simulink model "consistency"  (R2021a)
settings: Solver=VariableStepAuto  StartTime=0.0001  StopTime=180  FixedStep=0.01  RelTol=1e-6  AbsTol=1e-6
values from neighbouring files (symbols this model uses):
  A = kron(D,kron(B3,(B2*k1+B1*B2')))-kron(L,kron(B3,B2*k2))    [init.m]    (also in main.m)
  A_xi = kron(B3,B2*k1+B1*B2')    [init.m]    (also in main.m)
  B_h = kron(D,kron(B3,B2*k1))-kron(L,kron(B3,B2*k2))    [init.m]    (also in main.m)
  B_hv = kron(D,kron(B3,B2))    [init.m]    (also in main.m)
  B_xi = kron(VV(1,:),kron(B3,B1))    [init.m]    (also in main.m)
  theta0 = [theta10;theta20;theta30;theta40;theta50]    [init.m]    (also in main.m)
  xi0 = kron(VV(1,:),kron(B3,B3))*(theta0-ht0)    [init.m]    (also in main.m)
undefined symbols (not defined in the file or in its folder): dfcn_ht, fcn_ht, fcn_xi
settings Model: Creator=xxx  LastModifiedBy=Alpha
settings SolverCC: AutoScaleAbsTol=off  AlgebraicLoopSolver=TrustRegion
settings DataIOCC: ReturnWorkspaceOutputs=off
settings DebuggingCC: SFMachineParentedDataDiag=warning  ArithmeticOperatorsInVariantConditions=warning
settings SFSimCC: SimUseLocalCustomCode=off  CustomCodeUndefinedFunction=UseInterfaceOnly
settings RTWCC: RTWUseLocalCustomCode=off
settings CodeAppCC: StateflowObjectComments=on

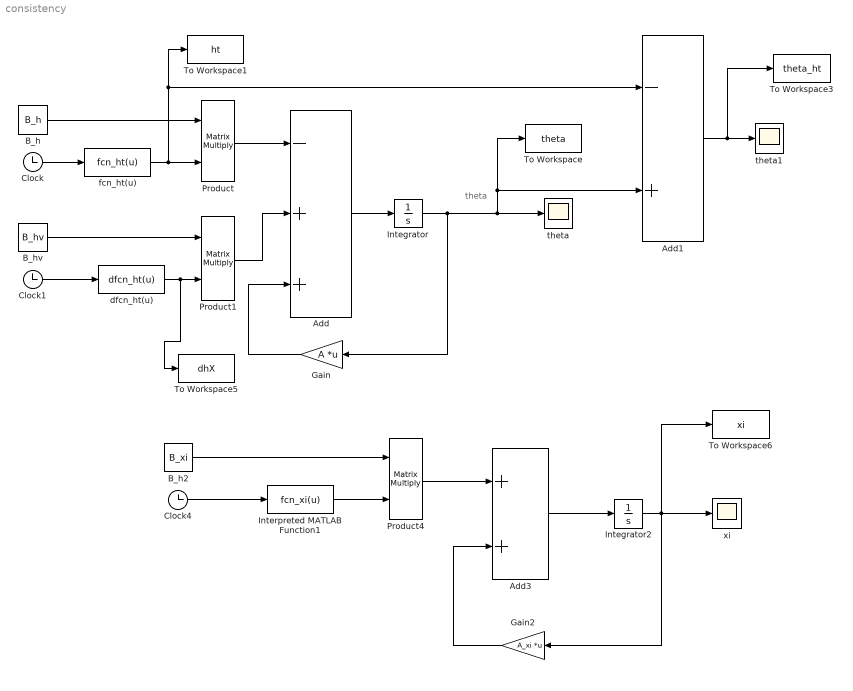
== system consistency ==
  note: theta
  Add : Sum  Inputs=-++
  Add1 : Sum  Inputs=-+
  Add3 : Sum
  B_h : Constant  Value=B_h
  B_h2 : Constant  Value=B_xi
  B_hv : Constant  Value=B_hv
  Clock : Clock
  Clock1 : Clock
  Clock4 : Clock
  Gain : Gain  Gain=A  Multiplication=Matrix(K*u)
  Gain2 : Gain  Gain=A_xi  Multiplication=Matrix(K*u)
  Integrator : Integrator  InitialCondition=theta0
  Integrator2 : Integrator  InitialCondition=xi0
  Interpreted MATLAB Function1 : MATLABFcn  MATLABFcn=fcn_xi(u)
  Product : Product  Multiplication=Matrix(*)
  Product1 : Product  Multiplication=Matrix(*)
  Product4 : Product  Multiplication=Matrix(*)
  To Workspace : ToWorkspace  VariableName=theta  SampleTime=-1
      settings: Save2DSignal=2-D array (concatenate along first dimension)
  To Workspace1 : ToWorkspace  VariableName=ht  SampleTime=-1
      settings: Save2DSignal=2-D array (concatenate along first dimension)
  To Workspace3 : ToWorkspace  VariableName=theta_ht  SampleTime=-1
      settings: Save2DSignal=2-D array (concatenate along first dimension)
  To Workspace5 : ToWorkspace  VariableName=dhX  SampleTime=-1
      settings: Save2DSignal=2-D array (concatenate along first dimension)
  To Workspace6 : ToWorkspace  VariableName=xi  SampleTime=-1
      settings: Save2DSignal=2-D array (concatenate along first dimension)
  dfcn_ht(u) : MATLABFcn  MATLABFcn=dfcn_ht(u)
  fcn_ht(u) : MATLABFcn  MATLABFcn=fcn_ht(u)
  theta : Scope
  theta1 : Scope
  xi : Scope
  wires:
  Add/1 -> Integrator/1
  Integrator/1 -> theta/1, Add1/2, To Workspace/1, Gain/1
  Gain/1 -> Add/3
  Clock/1 -> fcn_ht(u)/1
  fcn_ht(u)/1 -> To Workspace1/1, Add1/1, Product/2
  B_h/1 -> Product/1
  Clock1/1 -> dfcn_ht(u)/1
  dfcn_ht(u)/1 -> To Workspace5/1, Product1/2
  B_hv/1 -> Product1/1
  Add1/1 -> To Workspace3/1, theta1/1
  Add3/1 -> Integrator2/1
  Product4/1 -> Add3/1
  Interpreted MATLAB Function1/1 -> Product4/2
  B_h2/1 -> Product4/1
  Clock4/1 -> Interpreted MATLAB Function1/1
  Gain2/1 -> Add3/2
  Integrator2/1 -> To Workspace6/1, xi/1, Gain2/1
  Product/1 -> Add/1
  Product1/1 -> Add/2
